simulink model "HCSG_v1"  (R2018a)
settings: Solver=ode23tb  StartTime=0.0  StopTime=10000  MaxStep=0.1  RelTol=1e-3
values from neighbouring files (symbols this model uses):
  a_12 = h_wsc*pi*R_i/a_2    (= 0.891425789979)    [MSDR_parameters.m]
  a_4 = h_pw*pi*R_o/a_1    (= 0.0704483418498)    [MSDR_parameters.m]
  a_51 = Cp_p*W_p0/a_1    (= 1.13472152802)    [MSDR_parameters.m]
  a_53 = Cp_p*W_p2/a_1    (= 1.13472152802)    [MSDR_parameters.m]
  a_55 = Cp_p*W_p4/a_1    (= 1.13472152802)    [MSDR_parameters.m]
  a_6 = h_pw*pi*R_o/a_2    (= 1.27597922538)    [MSDR_parameters.m]
  a_7 = h_wb*pi*R_i/a_2    (= 1.41919299911)    [MSDR_parameters.m]
  a_8 = h_ws*pi*R_i/a_2    (= 0.609419981706)    [MSDR_parameters.m]
  A_p = pi*Ro_hydraulic^2    (= 0.00176802680852)    [MSDR_parameters.m]
  A_s = pi*(Ri_hydraulic^2)    (= 0.000137678413088)    [MSDR_parameters.m]
  A_w = pi*(Ro_thermal^2 - Ri_thermal^2)    (= 0.000101751473661)    [MSDR_parameters.m]
  Cp_p = 5591.471400012e-6    (= 0.00559147140001)    [MSDR_parameters.m]
  Cp_s = Cp_s*1e-6    [MSDR_parameters.m]
  Cp_sc = 4697.58960001e-6    (= 0.00469758960001)    [MSDR_parameters.m]
  Cp_w = 456.361200001e-6    (= 0.000456361200001)    [MSDR_parameters.m]
  dHs_dPs = c(1)    [MSDR_parameters.m]
  h_pw = 9101.343578935e-6    (= 0.00910134357894)    [MSDR_parameters.m]
  h_wb = 13349.334646671e-6    (= 0.0133493346467)    [MSDR_parameters.m]
  h_ws = 5732.378387768e-6    (= 0.00573237838777)    [MSDR_parameters.m]
  h_wsc = 8385.005556375e-6    (= 0.00838500555638)    [MSDR_parameters.m]
  K_1 = K_5    [MSDR_parameters.m]
  K_4 = b(1)    [MSDR_parameters.m]
  K_5 = a(1)    [MSDR_parameters.m]
  K_b = 12.834854076292217    (= 12.8348540763)    [MSDR_parameters.m]
  K_sc = -17.615718797133468    (= -17.6157187971)    [MSDR_parameters.m]
  L = 32    [MSDR_parameters.m]
  L_b = 21.5    [MSDR_parameters.m]
  L_s = L - L_b - L_sc    (= 6)    [MSDR_parameters.m]
  L_sc = 4.5    [MSDR_parameters.m]
  M_stm = 0.018    [MSDR_parameters.m]
  N = 820    [MSDR_parameters.m]
  P_s = P_s    (= 5.8)    [MSDR_parameters.m]
  P_sat = (5.8 + deltaP)    (= 6)    [MSDR_parameters.m]
  P_sc = P_s    (= 5.8)    [MSDR_parameters.m]
  P_set = P_s    (= 5.8)    [MSDR_parameters.m]
  R = 8.314462E-6    (= 8.314462e-06)    [MSDR_parameters.m]
  R_i = Ri_thermal    (= 0.00662)    [MSDR_parameters.m]
  R_o = Ro_thermal    (= 0.00873)    [MSDR_parameters.m]
  rho_p = 716.826235984    [MSDR_parameters.m]
  rho_s = 1/vss    [MSDR_parameters.m]
  rho_sc = (rho_fw + rho_f)/2    (= 789.870428969)    [MSDR_parameters.m]
  rho_w = 8425.711734699    (= 8425.7117347)    [MSDR_parameters.m]
  T_fw = 224    [MSDR_parameters.m]
  T_p1 = Tp10(end)    [MSDR_parameters.m]
  T_p2 = Tp20(end)    [MSDR_parameters.m]
  T_p3 = Tp30(end)    [MSDR_parameters.m]
  T_p4 = Tp40(end)    [MSDR_parameters.m]
  T_p5 = Tp50(end)    [MSDR_parameters.m]
  T_p6 = Tp60(end)    [MSDR_parameters.m]
  T_pin = 328.4    [MSDR_parameters.m]
  T_s1 = Ts10(end)    [MSDR_parameters.m]
  T_s2 = Ts20(end)    [MSDR_parameters.m]
  T_sc2 = Tsc20(end)    [MSDR_parameters.m]
  T_w1 = Tw10(end)    [MSDR_parameters.m]
  T_w2 = Tw20(end)    [MSDR_parameters.m]
  T_w3 = Tw30(end)    [MSDR_parameters.m]
  T_w4 = Tw40(end)    [MSDR_parameters.m]
  T_w5 = Tw50(end)    [MSDR_parameters.m]
  T_w6 = Tw60(end)    [MSDR_parameters.m]
  U_wb = 2*pi*R_i    (= 0.0415946867335)    [MSDR_parameters.m]
  U_ws = 2*pi*R_i    (= 0.0415946867335)    [MSDR_parameters.m]
  U_wsc = 2*pi*R_i    (= 0.0415946867335)    [MSDR_parameters.m]
  W_fw = W_sec    (= 0.0766463414634)    [MSDR_parameters.m]
  W_p0 = W_p    (= 0.719054878049)    [MSDR_parameters.m]
  X_4 = b(2)    [MSDR_parameters.m]
  X_5 = a(2)    [MSDR_parameters.m]
  Z_ss = 0.76634    [MSDR_parameters.m]
settings Model: Creator=viikr  LastModifiedBy=Vikram Singh

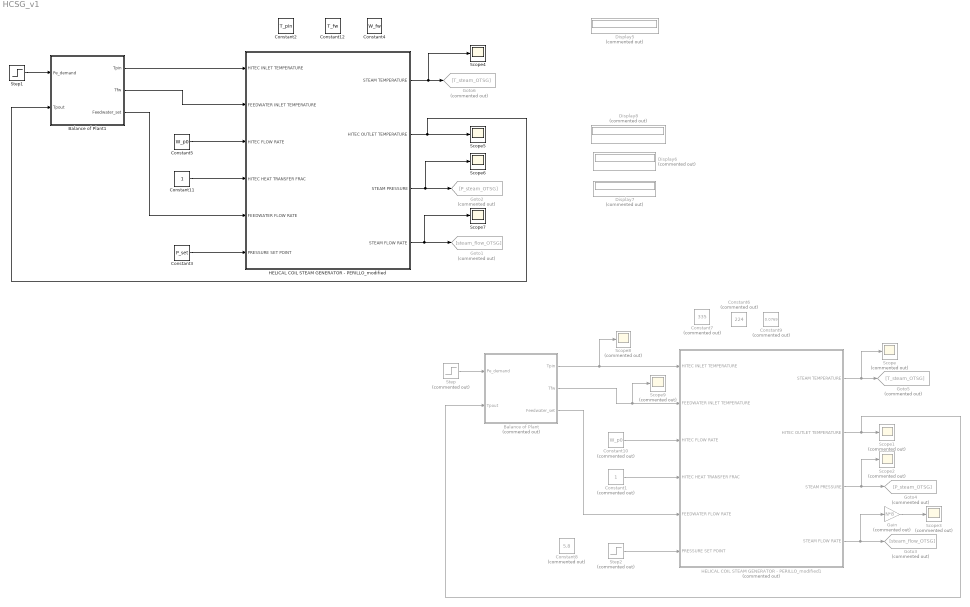
== system HCSG_v1 ==
  Balance of Plant : Subsystem  Commented=on
  Balance of Plant1 : Subsystem
  Constant1 : Constant  Commented=on
  Constant10 : Constant  Commented=on  Value=W_p0
  Constant11 : Constant
  Constant12 : Constant  Value=T_fw
  Constant2 : Constant  Value=T_pin
  Constant3 : Constant  Value=P_set
  Constant4 : Constant  Value=W_fw
  Constant5 : Constant  Value=W_p0
  Constant6 : Constant  Commented=on  Value=224
  Constant7 : Constant  Commented=on  Value=335
  Constant8 : Constant  Commented=on  Value=5.8
  Constant9 : Constant  Commented=on  Value=0.0769
  Display{5..8} (4 alike) : Display  Commented=on
  Gain : Gain  Commented=on  Gain=N*8
  Goto1 : Goto  Commented=on  GotoTag=steam_flow_OTSG
  Goto2 : Goto  Commented=on  GotoTag=P_steam_OTSG
  Goto3 : Goto  Commented=on  GotoTag=steam_flow_OTSG
  Goto4 : Goto  Commented=on  GotoTag=P_steam_OTSG
  Goto5 : Goto  Commented=on  GotoTag=T_steam_OTSG
  Goto6 : Goto  Commented=on  GotoTag=T_steam_OTSG
  HELICAL COIL STEAM GENERATOR - PERILLO_modified : Subsystem
  HELICAL COIL STEAM GENERATOR - PERILLO_modified1 : Subsystem  Commented=on
  Scope{,1..3,8..9} (6 alike) : Scope  Commented=on
  Scope{4..7} (4 alike) : Scope
  Step : Step  Commented=on  Time=2500  Before=100  After=95  SampleTime=0
  Step1 : Step  Time=2500  Before=100  After=95  SampleTime=0
  Step2 : Step  Commented=on  Time=5000  Before=5.8  After=5.9  SampleTime=0
  wires:
  HELICAL COIL STEAM GENERATOR - PERILLO_modified/3(STEAM PRESSURE) -> Scope6/1, Goto2/1
  HELICAL COIL STEAM GENERATOR - PERILLO_modified/1(STEAM TEMPERATURE) -> Scope4/1, Goto6/1
  HELICAL COIL STEAM GENERATOR - PERILLO_modified/4(STEAM FLOW RATE) -> Scope7/1, Goto1/1
  Constant11/1 -> HELICAL COIL STEAM GENERATOR - PERILLO_modified/4(HITEC HEAT TRANSFER FRAC)
  Constant3/1 -> HELICAL COIL STEAM GENERATOR - PERILLO_modified/6(PRESSURE SET POINT)
  HELICAL COIL STEAM GENERATOR - PERILLO_modified1/1(STEAM TEMPERATURE) -> Scope/1, Goto5/1
  Constant1/1 -> HELICAL COIL STEAM GENERATOR - PERILLO_modified1/4(HITEC HEAT TRANSFER FRAC)
  Constant10/1 -> HELICAL COIL STEAM GENERATOR - PERILLO_modified1/3(HITEC FLOW RATE)
  HELICAL COIL STEAM GENERATOR - PERILLO_modified1/3(STEAM PRESSURE) -> Scope2/1, Goto4/1
  HELICAL COIL STEAM GENERATOR - PERILLO_modified1/2(HITEC OUTLET TEMPERATURE) -> Scope1/1, Balance of Plant/2(Tpout)
  HELICAL COIL STEAM GENERATOR - PERILLO_modified1/4(STEAM FLOW RATE) -> Gain/1, Goto3/1
  Balance of Plant/1(Tpin) -> Scope8/1, HELICAL COIL STEAM GENERATOR - PERILLO_modified1/1(HITEC INLET TEMPERATURE)
  Balance of Plant/2(Tfw) -> Scope9/1, HELICAL COIL STEAM GENERATOR - PERILLO_modified1/2(FEEDWATER INLET TEMPERATURE)
  Balance of Plant/3(Feedwater_set) -> HELICAL COIL STEAM GENERATOR - PERILLO_modified1/5(FEEDWATER FLOW RATE)
  Step/1 -> Balance of Plant/1(Pe_demand)
  HELICAL COIL STEAM GENERATOR - PERILLO_modified/2(HITEC OUTLET TEMPERATURE) -> Balance of Plant1/2(Tpout), Scope5/1
  Balance of Plant1/2(Tfw) -> HELICAL COIL STEAM GENERATOR - PERILLO_modified/2(FEEDWATER INLET TEMPERATURE)
  Balance of Plant1/3(Feedwater_set) -> HELICAL COIL STEAM GENERATOR - PERILLO_modified/5(FEEDWATER FLOW RATE)
  Balance of Plant1/1(Tpin) -> HELICAL COIL STEAM GENERATOR - PERILLO_modified/1(HITEC INLET TEMPERATURE)
  Step1/1 -> Balance of Plant1/1(Pe_demand)
  Constant5/1 -> HELICAL COIL STEAM GENERATOR - PERILLO_modified/3(HITEC FLOW RATE)
  Step2/1 -> HELICAL COIL STEAM GENERATOR - PERILLO_modified1/6(PRESSURE SET POINT)
  Gain/1 -> Scope3/1

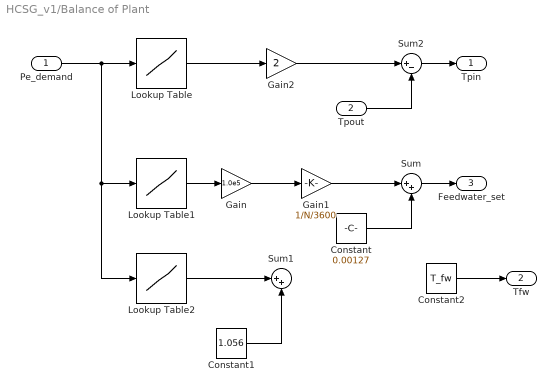
== system HCSG_v1/Balance of Plant ==
  Pe_demand : Inport
  Tpout : Inport  Port=2
  Constant : Constant  Value=0.00127
  Constant1 : Constant  Value=1.056
  Constant2 : Constant  Value=T_fw
  Gain : Gain  Gain=1.0e5
  Gain1 : Gain  Gain=1/N/3600
  Gain2 : Gain  Gain=2
  Lookup Table : Lookup  InputValues=[40, 60, 80, 90, 100]  Table="[304.8611, 306.4167,  308.2500, 309.0278,  310.0000]"
  Lookup Table1 : Lookup  InputValues=[40, 60, 80, 90, 100]  Table=[0.95708, 1.4016, 1.827977, 2.032094, 2.231674]
  Lookup Table2 : Lookup  InputValues=[40, 60, 80, 90, 100]  Table=[112.556, 156.61, 192.833, 208.556, 222.945]
  Sum : Sum  Inputs=|++
  Sum1 : Sum  Inputs=|++
  Sum2 : Sum  Inputs=|+-
  Tpin : Outport
  Tfw : Outport  Port=2
  Feedwater_set : Outport  Port=3
  wires:
  Pe_demand/1 -> Lookup Table1/1, Lookup Table2/1, Lookup Table/1
  Lookup Table/1 -> Gain2/1
  Lookup Table1/1 -> Gain/1
  Gain/1 -> Gain1/1
  Gain1/1 -> Sum/1
  Constant/1 -> Sum/2
  Sum/1 -> Feedwater_set/1
  Lookup Table2/1 -> Sum1/1
  Constant1/1 -> Sum1/2
  Gain2/1 -> Sum2/1
  Tpout/1 -> Sum2/2
  Sum2/1 -> Tpin/1
  Constant2/1 -> Tfw/1

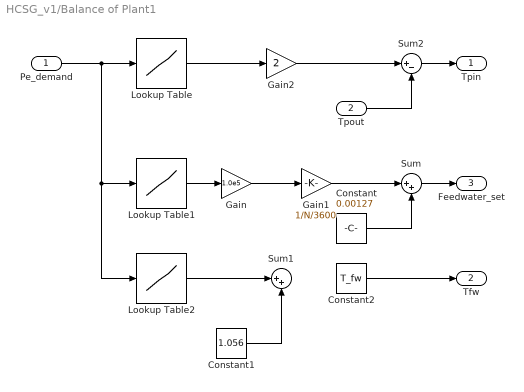
== system HCSG_v1/Balance of Plant1 ==
  Pe_demand : Inport
  Tpout : Inport  Port=2
  Constant : Constant  Value=0.00127
  Constant1 : Constant  Value=1.056
  Constant2 : Constant  Value=T_fw
  Gain : Gain  Gain=1.0e5
  Gain1 : Gain  Gain=1/N/3600
  Gain2 : Gain  Gain=2
  Lookup Table : Lookup  InputValues=[40, 60, 80, 90, 100]  Table="[304.8611, 306.4167,  308.2500, 309.0278,  310.0000]"
  Lookup Table1 : Lookup  InputValues=[40, 60, 80, 90, 100]  Table=[0.95708, 1.4016, 1.827977, 2.032094, 2.231674]
  Lookup Table2 : Lookup  InputValues=[40, 60, 80, 90, 100]  Table=[112.556, 156.61, 192.833, 208.556, 222.945]
  Sum : Sum  Inputs=|++
  Sum1 : Sum  Inputs=|++
  Sum2 : Sum  Inputs=|+-
  Tpin : Outport
  Tfw : Outport  Port=2
  Feedwater_set : Outport  Port=3
  wires:
  Pe_demand/1 -> Lookup Table1/1, Lookup Table2/1, Lookup Table/1
  Lookup Table/1 -> Gain2/1
  Lookup Table1/1 -> Gain/1
  Gain/1 -> Gain1/1
  Gain1/1 -> Sum/1
  Constant/1 -> Sum/2
  Sum/1 -> Feedwater_set/1
  Lookup Table2/1 -> Sum1/1
  Constant1/1 -> Sum1/2
  Gain2/1 -> Sum2/1
  Tpout/1 -> Sum2/2
  Sum2/1 -> Tpin/1
  Constant2/1 -> Tfw/1

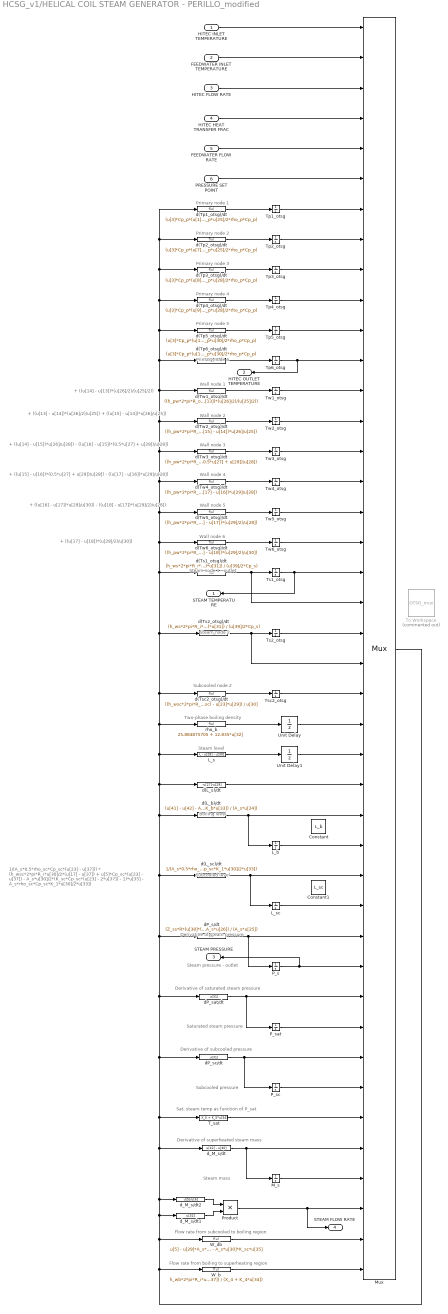
== system HCSG_v1/HELICAL COIL STEAM GENERATOR - PERILLO_modified ==
  note: + ((u[17] - u[18])*(u[29]/2)/u[30])
  note: + ((u[16] - u[17])*u[29]/u[30]) - ((u[18] - u[17])*(u[29]/2)/u[28])
  note: + ((u[15] - u[16])*(0.5*u[27] + u[29])/u[28]) - ((u[17] - u[16])*u[29]/u[28])
  note: + ((u[14] - u[15])*u[26]/u[28]) - ((u[16] - u[15])*(0.5*u[27] + u[29])/u[28])
  note: + ((u[13] - u[14])*(u[26]/2)/u[25]) + ((u[15] - u[14])*u[26]/u[25])
  note: + ((u[14] - u[13])*(u[26]/2)/(u[25]/2))
  note: 1/(A_s*0.5*rho_sc*Cp_sc*(u[23] - u[37])) * (h_wsc*2*pi*R_i*u[30]/2*(u[17] - u[37]) + u[5]*Cp_sc*(u[23] - u[37]) - A_s*u[30]/2*(K_sc*Cp_sc*(u[23] - 2*u[37]) - 1)*u[35] - A_s*rho_sc*Cp_sc*K_1*u[30]/2*u[33])
  note: Primary node 1
  note: Primary node 2
  note: Primary node 3
  note: Primary node 4
  note: Primary node 5
  note: Primary node 6
  note: Wall node 1
  note: Wall node 2
  note: Wall node 3
  note: Wall node 4
  note: Wall node 5
  note: Wall node 6
  note: Steam node 1 - outlet
  note: Steam level
  note: Boiling level
  note: Subcooled level
  note: Derivative of saturated steam pressure
  note: Sat. steam temp as function of P_sat
  note: Saturated steam pressure
  note: Subcooled pressure
  note: Derivative of steam pressure
  note: Derivative of subcooled pressure
  note: Steam pressure - outlet
  note: Subcooled node 2
  note: Steam node 2
  note: Two-phase boiling density
  note: Derivative of superheated steam mass
  note: Steam mass
  note: Flow rate from subcooled to boiling region
  note: Flow rate from boiling to superheating region
  HITEC INLET TEMPERATURE : Inport
  FEEDWATER INLET TEMPERATURE : Inport  Port=2
  HITEC FLOW RATE : Inport  Port=3
  HITEC HEAT TRANSFER FRAC : Inport  Port=4
  FEEDWATER FLOW RATE : Inport  Port=5
  PRESSURE SET POINT : Inport  Port=6
  Constant : Constant  Value=L_b
  Constant1 : Constant  Value=L_sc
  L_b : Integrator  InitialCondition=L_b
  L_s : Fcn  Expr=L - u[28] - u[30]
  L_sc : Integrator  InitialCondition=L_sc
  M_s : Integrator  InitialCondition=rho_s*A_s*L_s
  Mux : Mux  Inputs=42
      settings: DisplayOption=signals
  P_s : Integrator  InitialCondition=P_s
  P_sat : Integrator  InitialCondition=P_sat
  P_sc : Integrator  InitialCondition=P_sc
  Product : Product
  T_sat : Fcn  Expr=X_5 + K_5*u[34]
  To Workspace : ToWorkspace  Commented=on  VariableName=OTSG_mux  SampleTime=-1
      settings: Save2DSignal=2-D array (concatenate along first dimension)
  Tp1_otsg : Integrator  InitialCondition=T_p1
  Tp2_otsg : Integrator  InitialCondition=T_p2
  Tp3_otsg : Integrator  InitialCondition=T_p3
  Tp4_otsg : Integrator  InitialCondition=T_p4
  Tp5_otsg : Integrator  InitialCondition=T_p5
  Tp6_otsg : Integrator  InitialCondition=T_p6
  Ts1_otsg : Integrator  InitialCondition=T_s1
  Ts2_otsg : Integrator  InitialCondition=T_s2
  Tsc2_otsg : Integrator  InitialCondition=T_sc2
  Tw1_otsg : Integrator  InitialCondition=T_w1
  Tw2_otsg : Integrator  InitialCondition=T_w2
  Tw3_otsg : Integrator  InitialCondition=T_w3
  Tw4_otsg : Integrator  InitialCondition=T_w4
  Tw5_otsg : Integrator  InitialCondition=T_w5
  Tw6_otsg : Integrator  InitialCondition=T_w6
  Unit Delay : UnitDelay  InitialCondition=100  SampleTime=-1
  Unit Delay1 : UnitDelay  InitialCondition=L_s  SampleTime=-1
  W_b : Fcn  Expr=h_wb*2*pi*R_i*u[28]*(0.5*u[15] + 0.5*u[16] - u[37]) / (X_4 + K_4*u[34])
  W_db : Fcn  Expr=u[5] - u[29]*A_s*rho_sc - A_s*u[30]*K_sc*u[35]
  d(L_b)/dt : Fcn  Expr=(u[41] - u[42] - A_s*u[28]*K_b*u[33]) / (A_s*u[24])
  d(L_s)/dt : Fcn  Expr=-u[27]-u[29]
  d(L_sc)/dt : Fcn  Expr=1/(A_s*0.5*rho_sc*Cp_sc*(u[23] - u[37])) * (h_wsc*2*pi*R_i*u[30]/2*(u[17] - u[37]) + u[5]*Cp_sc*(u[23] - u[37]) - A_s*u[30]/2*(K_sc*Cp_sc*(u[23] - 2*u[37]) - 1)*u[35] - A_s*rho_sc*Cp_sc*K_1*u[30]/2*u[33])
  d(Tp1_otsg)/dt : Fcn  Expr=(u[3]*Cp_p*(u[1] - u[7]) + h_pw*2*pi*R_o*u[25]/2*(u[13] - u[7])) / (A_p*u[25]/2*rho_p*Cp_p)
  d(Tp2_otsg)/dt : Fcn  Expr=(u[3]*Cp_p*(u[7] - u[8]) + h_pw*2*pi*R_o*u[25]/2*(u[14] - u[8])) / (A_p*u[25]/2*rho_p*Cp_p)
  d(Tp3_otsg)/dt : Fcn  Expr=(u[3]*Cp_p*(u[8] - u[9]) + h_pw*2*pi*R_o*u[28]/2*(u[15] - u[9])) / (A_p*u[28]/2*rho_p*Cp_p)
  d(Tp4_otsg)/dt : Fcn  Expr=(u[3]*Cp_p*(u[9] - u[10]) + h_pw*2*pi*R_o*u[28]/2*(u[16] - u[10])) / (A_p*u[28]/2*rho_p*Cp_p)
  d(Tp5_otsg)/dt : Fcn  Expr=(u[3]*Cp_p*(u[10] - u[11]) + h_pw*2*pi*R_o*u[30]/2*(u[17] - u[11])) / (A_p*u[30]/2*rho_p*Cp_p)
  d(Tp6_otsg)/dt : Fcn  Expr=(u[3]*Cp_p*(u[11] - u[12]) + h_pw*2*pi*R_o*u[30]/2*(u[18] - u[12])) / (A_p*u[30]/2*rho_p*Cp_p)
  d(Ts1_otsg)/dt : Fcn  Expr="(h_ws*2*pi*R_i*u[25]/2*(u[13] - u[19]) + u[40]*Cp_s*(u[21] - u[19]) +  Cp_s*(u[21] - u[19])*u[38]/2 + (A_s*u[25]/2 - u[39]/2*dHs_dPs)*u[31]) / (u[39]/2*Cp_s)"
  d(Ts2_otsg)/dt : Fcn  Expr=(h_ws*2*pi*R_i*u[25]/2*(u[14] - u[21]) + u[42]*Cp_s*(u[37] - u[21]) + (A_s*u[25]/2 - u[39]/2*dHs_dPs)*u[31]) / (u[39]/2*Cp_s)
  d(Tsc2_otsg)/dt : Fcn  Expr=((h_wsc*2*pi*R_i*u[30]/2*(u[18] - u[23]) + Cp_sc*(u[5]*u[2] - (u[5] + u[41])*0.5*u[23]) + A_s*u[30]/2*u[35]) * 2/(A_s*rho_sc*Cp_sc) - u[23]*u[29]) / u[30]
  d(Tw1_otsg)/dt : Fcn  Expr=((h_pw*2*pi*R_o*u[25]/2*(u[7] - u[13]) + h_ws*2*pi*R_i*u[25]/2*(u[19] - u[13])) / (A_w*u[25]/2*rho_w*Cp_w)) + ((u[14] - u[13])*(u[26]/2)/(u[25]/2))
  d(Tw2_otsg)/dt : Fcn  Expr="((h_pw*2*pi*R_o*u[25]/2*(u[8] - u[14]) + h_ws*2*pi*R_i*u[25]/2*(u[21] - u[14])) / (A_w*u[25]/2*rho_w*Cp_w))  + ((u[13] - u[14])*(u[26]/2)/u[25]) + ((u[15] - u[14])*u[26]/u[25])"
  d(Tw3_otsg)/dt : Fcn  Expr="((h_pw*2*pi*R_o*u[28]/2*(u[9] - u[15]) + h_wb*2*pi*R_i*u[28]/2*(u[37] - u[15])) / (A_w*u[28]/2*rho_w*Cp_w))  + ((u[14] - u[15])*u[26]/u[28]) - ((u[16] - u[15])*(0.5*u[27] + u[29])/u[28])"
  d(Tw4_otsg)/dt : Fcn  Expr="((h_pw*2*pi*R_o*u[28]/2*(u[10] - u[16]) + h_wb*2*pi*R_i*u[28]/2*(u[37] - u[16])) / (A_w*u[28]/2*rho_w*Cp_w)) +  + ((u[15] - u[16])*(0.5*u[27] + u[29])/u[28]) - ((u[17] - u[16])*u[29]/u[28])"
  d(Tw5_otsg)/dt : Fcn  Expr="((h_pw*2*pi*R_o*u[30]/2*(u[11] - u[17]) + h_wsc*2*pi*R_i*u[30]/2*(u[37] - u[17])) / (A_w*u[30]/2*rho_w*Cp_w))  + ((u[16] - u[17])*u[29]/u[30]) - ((u[18] - u[17])*(u[29]/2)/u[28])"
  d(Tw6_otsg)/dt : Fcn  Expr="((h_pw*2*pi*R_o*u[30]/2*(u[12] - u[18]) + h_wsc*2*pi*R_i*u[30]/2*(u[23] - u[18])) / (A_w*u[30]/2*rho_w*Cp_w))  + ((u[17] - u[18])*(u[29]/2)/u[30])"
  dP_s/dt : Fcn  Expr=(Z_ss*R*(u[38]*(u[19] + u[21]) + u[39]*(u[20] + u[22]))/(2*M_stm) - u[32]*A_s*u[26]) / (A_s*u[25])
  dP_sat/dt : Fcn  Expr=u[31]
  dP_sc/dt : Fcn  Expr=u[31]
  d_M_s/dt : Fcn  Expr=u[42] - u[40]
  d_M_s/dt1 : Fcn  Expr=u[32]
  d_M_s/dt2 : Fcn  Expr=u[5]/u[6]
  rho_b : Fcn  Expr=25.884875705 + 12.835*u[32]
  STEAM TEMPERATURE : Outport
  HITEC OUTLET TEMPERATURE : Outport  Port=2
  STEAM PRESSURE : Outport  Port=3
  STEAM FLOW RATE : Outport  Port=4
  wires:
  FEEDWATER INLET TEMPERATURE/1 -> Mux/2
  d(Tp1_otsg)/dt/1 -> Tp1_otsg/1
  HITEC INLET TEMPERATURE/1 -> Mux/1
  HITEC FLOW RATE/1 -> Mux/3
  HITEC HEAT TRANSFER FRAC/1 -> Mux/4
  FEEDWATER FLOW RATE/1 -> Mux/5
  PRESSURE SET POINT/1 -> Mux/6
  Tp1_otsg/1 -> Mux/7
  Tp2_otsg/1 -> Mux/8
  d(Tp2_otsg)/dt/1 -> Tp2_otsg/1
  Tp3_otsg/1 -> Mux/9
  d(Tp3_otsg)/dt/1 -> Tp3_otsg/1
  Tp4_otsg/1 -> Mux/10
  d(Tp4_otsg)/dt/1 -> Tp4_otsg/1
  Tp5_otsg/1 -> Mux/11
  d(Tp5_otsg)/dt/1 -> Tp5_otsg/1
  d(Tp6_otsg)/dt/1 -> Tp6_otsg/1
  Tp6_otsg/1 -> HITEC OUTLET TEMPERATURE/1, Mux/12
  Tw1_otsg/1 -> Mux/13
  d(Tw1_otsg)/dt/1 -> Tw1_otsg/1
  d(Tw2_otsg)/dt/1 -> Tw2_otsg/1
  Tw2_otsg/1 -> Mux/14
  Tw3_otsg/1 -> Mux/15
  d(Tw3_otsg)/dt/1 -> Tw3_otsg/1
  d(Tw4_otsg)/dt/1 -> Tw4_otsg/1
  Tw4_otsg/1 -> Mux/16
  Tw5_otsg/1 -> Mux/17
  d(Tw5_otsg)/dt/1 -> Tw5_otsg/1
  d(Tw6_otsg)/dt/1 -> Tw6_otsg/1
  Tw6_otsg/1 -> Mux/18
  Ts1_otsg/1 -> STEAM TEMPERATURE/1, Mux/19
  dP_sc/dt/1 -> Mux/35, P_sc/1
  P_sat/1 -> Mux/34
  P_sc/1 -> Mux/36
  dP_sat/dt/1 -> Mux/33, P_sat/1
  T_sat/1 -> Mux/37
  dP_s/dt/1 -> Mux/31, P_s/1
  Tsc2_otsg/1 -> Mux/23
  d(Tsc2_otsg)/dt/1 -> Tsc2_otsg/1
  Ts2_otsg/1 -> Mux/21
  rho_b/1 -> Unit Delay/1
  d(Ts1_otsg)/dt/1 -> Mux/20, Ts1_otsg/1
  d(Ts2_otsg)/dt/1 -> Mux/22, Ts2_otsg/1
  M_s/1 -> Mux/39
  d_M_s/dt/1 -> Mux/38, M_s/1
  d(L_b)/dt/1 -> Mux/27, L_b/1
  d(L_sc)/dt/1 -> Mux/29, L_sc/1
  Product/1 -> Mux/40, STEAM FLOW RATE/1
  L_s/1 -> Unit Delay1/1
  d(L_s)/dt/1 -> Mux/26
  P_s/1 -> Mux/32, STEAM PRESSURE/1
  W_db/1 -> Mux/41
  W_b/1 -> Mux/42
  Mux/1 -> W_b/1, W_db/1, d_M_s/dt/1, T_sat/1, dP_sc/dt/1, dP_sat/dt/1, dP_s/dt/1, d(L_sc)/dt/1, d(L_b)/dt/1, d(L_s)/dt/1, L_s/1, rho_b/1, d(Tsc2_otsg)/dt/1, d(Ts2_otsg)/dt/1, d(Ts1_otsg)/dt/1, d(Tw6_otsg)/dt/1, d(Tw5_otsg)/dt/1, d(Tw4_otsg)/dt/1, d(Tw3_otsg)/dt/1, d(Tw2_otsg)/dt/1, d(Tw1_otsg)/dt/1, d(Tp6_otsg)/dt/1, d(Tp5_otsg)/dt/1, d(Tp4_otsg)/dt/1, d(Tp3_otsg)/dt/1, d(Tp2_otsg)/dt/1, d(Tp1_otsg)/dt/1, d_M_s/dt2/1, d_M_s/dt1/1
  d_M_s/dt2/1 -> Product/1
  d_M_s/dt1/1 -> Product/2
  L_b/1 -> Mux/28
  L_sc/1 -> Mux/30
  Unit Delay/1 -> Mux/24
  Unit Delay1/1 -> Mux/25

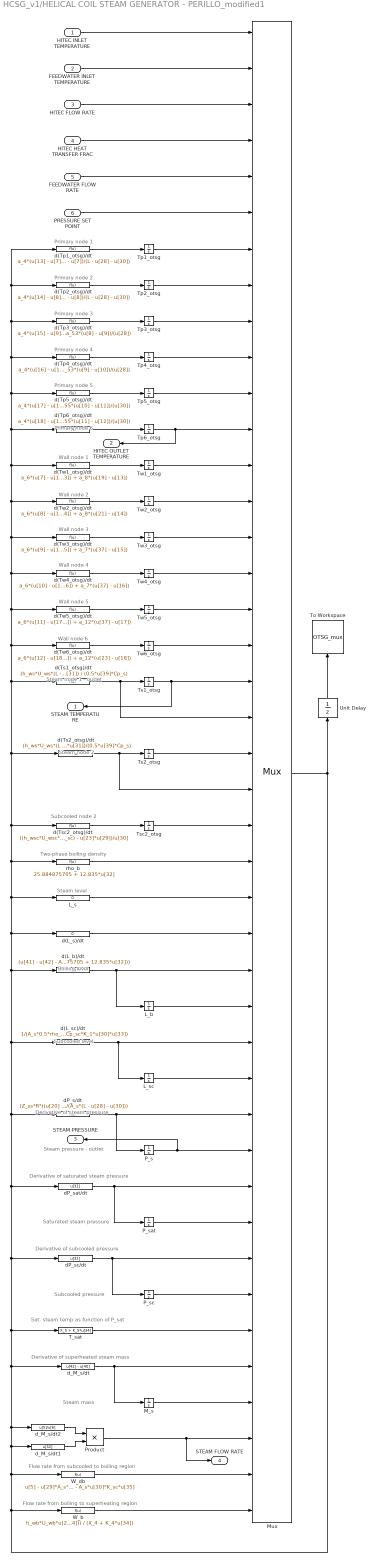
== system HCSG_v1/HELICAL COIL STEAM GENERATOR - PERILLO_modified1 ==
  note: Primary node 1
  note: Primary node 2
  note: Primary node 3
  note: Primary node 4
  note: Primary node 5
  note: Primary node 6
  note: Wall node 1
  note: Wall node 2
  note: Wall node 3
  note: Wall node 4
  note: Wall node 5
  note: Wall node 6
  note: Steam node 1 - outlet
  note: Steam level
  note: Boiling level
  note: Subcooled level
  note: Derivative of saturated steam pressure
  note: Sat. steam temp as function of P_sat
  note: Saturated steam pressure
  note: Subcooled pressure
  note: Derivative of steam pressure
  note: Derivative of subcooled pressure
  note: Steam pressure - outlet
  note: Subcooled node 2
  note: Steam node 2
  note: Two-phase boiling density
  note: Derivative of superheated steam mass
  note: Steam mass
  note: Flow rate from subcooled to boiling region
  note: Flow rate from boiling to superheating region
  HITEC INLET TEMPERATURE : Inport
  FEEDWATER INLET TEMPERATURE : Inport  Port=2
  HITEC FLOW RATE : Inport  Port=3
  HITEC HEAT TRANSFER FRAC : Inport  Port=4
  FEEDWATER FLOW RATE : Inport  Port=5
  PRESSURE SET POINT : Inport  Port=6
  L_b : Integrator  InitialCondition=L_b
  L_s : Fcn  Expr=0
  L_sc : Integrator  InitialCondition=L_sc
  M_s : Integrator  InitialCondition=rho_s*A_s*L_s
  Mux : Mux  Inputs=42
      settings: DisplayOption=signals
  P_s : Integrator  InitialCondition=P_s
  P_sat : Integrator  InitialCondition=P_sat
  P_sc : Integrator  InitialCondition=P_sc
  Product : Product
  T_sat : Fcn  Expr=X_5 + K_5*u[34]
  To Workspace : ToWorkspace  VariableName=OTSG_mux  SampleTime=-1
      settings: Save2DSignal=2-D array (concatenate along first dimension)
  Tp1_otsg : Integrator  InitialCondition=T_p1
  Tp2_otsg : Integrator  InitialCondition=T_p2
  Tp3_otsg : Integrator  InitialCondition=T_p3
  Tp4_otsg : Integrator  InitialCondition=T_p4
  Tp5_otsg : Integrator  InitialCondition=T_p5
  Tp6_otsg : Integrator  InitialCondition=T_p6
  Ts1_otsg : Integrator  InitialCondition=T_s1
  Ts2_otsg : Integrator  InitialCondition=T_s2
  Tsc2_otsg : Integrator  InitialCondition=T_sc2
  Tw1_otsg : Integrator  InitialCondition=T_w1
  Tw2_otsg : Integrator  InitialCondition=T_w2
  Tw3_otsg : Integrator  InitialCondition=T_w3
  Tw4_otsg : Integrator  InitialCondition=T_w4
  Tw5_otsg : Integrator  InitialCondition=T_w5
  Tw6_otsg : Integrator  InitialCondition=T_w6
  Unit Delay : UnitDelay  SampleTime=-1
  W_b : Fcn  Expr=h_wb*U_wb*u[28]*(0.5*u[15] + 0.5*u[16] - (X_5 + K_5*u[34])) / (X_4 + K_4*u[34])
  W_db : Fcn  Expr=u[5] - u[29]*A_s*rho_sc - A_s*u[30]*K_sc*u[35]
  d(L_b)/dt : Fcn  Expr=(u[41] - u[42] - A_s*u[28]*K_b*u[35]) / (A_s*(25.884875705 + 12.835*u[32]))
  d(L_s)/dt : Fcn  Expr=0
  d(L_sc)/dt : Fcn  Expr=1/(A_s*0.5*rho_sc*Cp_sc*(u[23] - u[37])) * (h_wsc*U_wsc*0.5*u[30]*(u[17] - u[37]) + u[5]*Cp_sc*(u[23] - u[37]) - 0.5*A_s*u[30]*(K_sc*Cp_sc*(u[23] - 2*u[37]) - 1)*u[35] - 0.5*A_s*rho_sc*Cp_sc*K_1*u[30]*u[33])
  d(Tp1_otsg)/dt : Fcn  Expr=a_4*(u[13] - u[7]) + a_51*(u[1] - u[7])/(L - u[28] - u[30])
  d(Tp2_otsg)/dt : Fcn  Expr=a_4*(u[14] - u[8]) + a_51*(u[7] - u[8])/(L - u[28] - u[30])
  d(Tp3_otsg)/dt : Fcn  Expr=a_4*(u[15] - u[9]) + a_53*(u[8] - u[9])/(u[28])
  d(Tp4_otsg)/dt : Fcn  Expr=a_4*(u[16] - u[10]) + a_53*(u[9] - u[10])/(u[28])
  d(Tp5_otsg)/dt : Fcn  Expr=a_4*(u[17] - u[11]) + a_55*(u[10] - u[11])/(u[30])
  d(Tp6_otsg)/dt : Fcn  Expr=a_4*(u[18] - u[12]) + a_55*(u[11] - u[12])/(u[30])
  d(Ts1_otsg)/dt : Fcn  Expr=(h_ws*U_ws*(L - u[28] - u[30])*0.5*(u[13] - u[19]) + u[40]*Cp_s*(u[21] - u[19]) + Cp_s*(u[21] - u[19])*0.5*u[38] - (0.5*u[39]*dHs_dPs - A_s*0.5*(L - u[28] - u[30]))*u[31]) / (0.5*u[39]*Cp_s)
  d(Ts2_otsg)/dt : Fcn  Expr=(h_ws*U_ws*(L - u[28] - u[30])*0.5*(u[14] - u[21]) + (h_wb*U_wb*u[28]*(0.5*u[15] + 0.5*u[16] - u[37])/(X_4 + K_4*u[34]))*Cp_s*(u[37] - u[21]) - (0.5*u[39]*dHs_dPs - A_s*0.5*(L - u[28] - u[30]))*u[31])/(0.5*u[39]*Cp_s)
  d(Tsc2_otsg)/dt : Fcn  Expr=((h_wsc*U_wsc*0.5*u[30]*(u[18] - u[23]) + Cp_sc*(u[5]*u[2] - (0.5*(u[5] + u[5] - rho_sc*A_s*u[29] - A_s*u[30]*K_sc*u[35]))*u[23]) + 0.5*A_s*u[30]*u[35]) * 2/(A_s*rho_sc*Cp_sc) - u[23]*u[29])/u[30]
  d(Tw1_otsg)/dt : Fcn  Expr=a_6*(u[7] - u[13]) + a_8*(u[19] - u[13])
  d(Tw2_otsg)/dt : Fcn  Expr=a_6*(u[8] - u[14]) + a_8*(u[21] - u[14])
  d(Tw3_otsg)/dt : Fcn  Expr=a_6*(u[9] - u[15]) + a_7*(u[37] - u[15])
  d(Tw4_otsg)/dt : Fcn  Expr=a_6*(u[10] - u[16]) + a_7*(u[37] - u[16])
  d(Tw5_otsg)/dt : Fcn  Expr=a_6*(u[11] - u[17]) + a_12*(u[37] - u[17])
  d(Tw6_otsg)/dt : Fcn  Expr=a_6*(u[12] - u[18]) + a_12*(u[23] - u[18])
  dP_s/dt : Fcn  Expr=(Z_ss*R*((u[20] + u[22])*u[39] + (u[19] + u[21])*u[38])/(2*M_stm) - u[32]*A_s*(-u[29]-u[27]))/(A_s*(L - u[28] - u[30]))
  dP_sat/dt : Fcn  Expr=u[31]
  dP_sc/dt : Fcn  Expr=u[31]
  d_M_s/dt : Fcn  Expr=u[42] - u[40]
  d_M_s/dt1 : Fcn  Expr=u[32]
  d_M_s/dt2 : Fcn  Expr=u[5]/u[6]
  rho_b : Fcn  Expr=25.884875705 + 12.835*u[32]
  STEAM TEMPERATURE : Outport
  HITEC OUTLET TEMPERATURE : Outport  Port=2
  STEAM PRESSURE : Outport  Port=3
  STEAM FLOW RATE : Outport  Port=4
  wires:
  FEEDWATER INLET TEMPERATURE/1 -> Mux/2
  d(Tp1_otsg)/dt/1 -> Tp1_otsg/1
  HITEC INLET TEMPERATURE/1 -> Mux/1
  HITEC FLOW RATE/1 -> Mux/3
  HITEC HEAT TRANSFER FRAC/1 -> Mux/4
  FEEDWATER FLOW RATE/1 -> Mux/5
  PRESSURE SET POINT/1 -> Mux/6
  Tp1_otsg/1 -> Mux/7
  Tp2_otsg/1 -> Mux/8
  d(Tp2_otsg)/dt/1 -> Tp2_otsg/1
  Tp3_otsg/1 -> Mux/9
  d(Tp3_otsg)/dt/1 -> Tp3_otsg/1
  Tp4_otsg/1 -> Mux/10
  d(Tp4_otsg)/dt/1 -> Tp4_otsg/1
  Tp5_otsg/1 -> Mux/11
  d(Tp5_otsg)/dt/1 -> Tp5_otsg/1
  d(Tp6_otsg)/dt/1 -> Tp6_otsg/1
  Tp6_otsg/1 -> HITEC OUTLET TEMPERATURE/1, Mux/12
  Tw1_otsg/1 -> Mux/13
  d(Tw1_otsg)/dt/1 -> Tw1_otsg/1
  d(Tw2_otsg)/dt/1 -> Tw2_otsg/1
  Tw2_otsg/1 -> Mux/14
  Tw3_otsg/1 -> Mux/15
  d(Tw3_otsg)/dt/1 -> Tw3_otsg/1
  d(Tw4_otsg)/dt/1 -> Tw4_otsg/1
  Tw4_otsg/1 -> Mux/16
  Tw5_otsg/1 -> Mux/17
  d(Tw5_otsg)/dt/1 -> Tw5_otsg/1
  d(Tw6_otsg)/dt/1 -> Tw6_otsg/1
  Tw6_otsg/1 -> Mux/18
  Ts1_otsg/1 -> STEAM TEMPERATURE/1, Mux/19
  P_sat/1 -> Mux/34
  P_sc/1 -> Mux/36
  T_sat/1 -> Mux/37
  Tsc2_otsg/1 -> Mux/23
  d(Tsc2_otsg)/dt/1 -> Tsc2_otsg/1
  Ts2_otsg/1 -> Mux/21
  rho_b/1 -> Mux/24
  d(Ts1_otsg)/dt/1 -> Mux/20, Ts1_otsg/1
  d(Ts2_otsg)/dt/1 -> Mux/22, Ts2_otsg/1
  M_s/1 -> Mux/39
  d_M_s/dt/1 -> Mux/38, M_s/1
  d(L_b)/dt/1 -> Mux/27, L_b/1
  d(L_sc)/dt/1 -> Mux/29, L_sc/1
  Product/1 -> Mux/40, STEAM FLOW RATE/1
  L_s/1 -> Mux/25
  d(L_s)/dt/1 -> Mux/26
  P_s/1 -> Mux/32, STEAM PRESSURE/1
  W_db/1 -> Mux/41
  W_b/1 -> Mux/42
  Mux/1 -> Unit Delay/1, W_b/1, W_db/1, d_M_s/dt/1, T_sat/1, dP_sc/dt/1, dP_sat/dt/1, dP_s/dt/1, d(L_sc)/dt/1, d(L_b)/dt/1, d(L_s)/dt/1, L_s/1, rho_b/1, d(Tsc2_otsg)/dt/1, d(Ts2_otsg)/dt/1, d(Ts1_otsg)/dt/1, d(Tw6_otsg)/dt/1, d(Tw5_otsg)/dt/1, d(Tw4_otsg)/dt/1, d(Tw3_otsg)/dt/1, d(Tw2_otsg)/dt/1, d(Tw1_otsg)/dt/1, d(Tp6_otsg)/dt/1, d(Tp5_otsg)/dt/1, d(Tp4_otsg)/dt/1, d(Tp3_otsg)/dt/1, d(Tp2_otsg)/dt/1, d(Tp1_otsg)/dt/1, d_M_s/dt2/1, d_M_s/dt1/1
  d_M_s/dt2/1 -> Product/1
  d_M_s/dt1/1 -> Product/2
  L_b/1 -> Mux/28
  L_sc/1 -> Mux/30
  dP_s/dt/1 -> Mux/31, P_s/1
  dP_sat/dt/1 -> Mux/33, P_sat/1
  dP_sc/dt/1 -> Mux/35, P_sc/1
  Unit Delay/1 -> To Workspace/1
